simulink model "SWC_HALOUT_type"  (R2021b)
settings: Solver=FixedStepDiscrete  StartTime=0.0  StopTime=10.0  FixedStep=0.005  RelTol=1e-3
values from neighbouring files (symbols this model uses):
  DTC_10020B = Simulink.Parameter    [DTC_Constant_Definition.m]
  DTC_10020C = Simulink.Parameter    [DTC_Constant_Definition.m]
  DTC_10020D = Simulink.Parameter    [DTC_Constant_Definition.m]
  DTC_10020E = Simulink.Parameter    [DTC_Constant_Definition.m]
  DTC_100210 = Simulink.Parameter    [DTC_Constant_Definition.m]
  DTC_100211 = Simulink.Parameter    [DTC_Constant_Definition.m]
  DTC_100212 = Simulink.Parameter    [DTC_Constant_Definition.m]
  DTC_100213 = Simulink.Parameter    [DTC_Constant_Definition.m]
  DTC_100214 = Simulink.Parameter    [DTC_Constant_Definition.m]
  DTC_100215 = Simulink.Parameter    [DTC_Constant_Definition.m]
  DTC_100216 = Simulink.Parameter    [DTC_Constant_Definition.m]
  DTC_100217 = Simulink.Parameter    [DTC_Constant_Definition.m]
  DTC_100218 = Simulink.Parameter    [DTC_Constant_Definition.m]
  DTC_100219 = Simulink.Parameter    [DTC_Constant_Definition.m]
  DTC_10021A = Simulink.Parameter    [DTC_Constant_Definition.m]
  DTC_10021B = Simulink.Parameter    [DTC_Constant_Definition.m]
  DTC_10021C = Simulink.Parameter    [DTC_Constant_Definition.m]
  DTC_10021D = Simulink.Parameter    [DTC_Constant_Definition.m]
  DTC_10021E = Simulink.Parameter    [DTC_Constant_Definition.m]
  DTC_100220 = Simulink.Parameter    [DTC_Constant_Definition.m]
  DTC_100221 = Simulink.Parameter    [DTC_Constant_Definition.m]
  DTC_100223 = Simulink.Parameter    [DTC_Constant_Definition.m]
  DTC_100224 = Simulink.Parameter    [DTC_Constant_Definition.m]
  DTC_100225 = Simulink.Parameter    [DTC_Constant_Definition.m]
  DTC_100226 = Simulink.Parameter    [DTC_Constant_Definition.m]
  DTC_100227 = Simulink.Parameter    [DTC_Constant_Definition.m]
  DTC_100242 = Simulink.Parameter    [DTC_Constant_Definition.m]
  DTC_100243 = Simulink.Parameter    [DTC_Constant_Definition.m]
  DTC_100244 = Simulink.Parameter    [DTC_Constant_Definition.m]
  DTC_100247 = Simulink.Parameter    [DTC_Constant_Definition.m]
  DTC_100248 = Simulink.Parameter    [DTC_Constant_Definition.m]
  DTC_100249 = Simulink.Parameter    [DTC_Constant_Definition.m]
  DTC_100250 = Simulink.Parameter    [DTC_Constant_Definition.m]
  DTC_100251 = Simulink.Parameter    [DTC_Constant_Definition.m]
  DTC_100252 = Simulink.Parameter    [DTC_Constant_Definition.m]
  DTC_100A10 = Simulink.Parameter    [DTC_Constant_Definition.m]
  DTC_100A12 = Simulink.Parameter    [DTC_Constant_Definition.m]
  DTC_100A16 = Simulink.Parameter    [DTC_Constant_Definition.m]
  DTC_100A17 = Simulink.Parameter    [DTC_Constant_Definition.m]
  DTC_100A18 = Simulink.Parameter    [DTC_Constant_Definition.m]
  DTC_100A19 = Simulink.Parameter    [DTC_Constant_Definition.m]
  DTC_500B01 = Simulink.Parameter    [DTC_Constant_Definition.m]
  DTC_500B02 = Simulink.Parameter    [DTC_Constant_Definition.m]
  DTC_500B03 = Simulink.Parameter    [DTC_Constant_Definition.m]
  DTC_500B04 = Simulink.Parameter    [DTC_Constant_Definition.m]
  DTC_500B05 = Simulink.Parameter    [DTC_Constant_Definition.m]
  DTC_500B06 = Simulink.Parameter    [DTC_Constant_Definition.m]
  DTC_500B07 = Simulink.Parameter    [DTC_Constant_Definition.m]
  DTC_500B08 = Simulink.Parameter    [DTC_Constant_Definition.m]
  DTC_500B09 = Simulink.Parameter    [DTC_Constant_Definition.m]
  DTC_500B0A = Simulink.Parameter    [DTC_Constant_Definition.m]
  DTC_500B0B = Simulink.Parameter    [DTC_Constant_Definition.m]
  DTC_500B0C = Simulink.Parameter    [DTC_Constant_Definition.m]
  DTC_500B0D = Simulink.Parameter    [DTC_Constant_Definition.m]
  DTC_500B0E = Simulink.Parameter    [DTC_Constant_Definition.m]
  DTC_500B0F = Simulink.Parameter    [DTC_Constant_Definition.m]
  DTC_500B10 = Simulink.Parameter    [DTC_Constant_Definition.m]
  DTC_90021F = Simulink.Parameter    [DTC_Constant_Definition.m]
  DTC_90022F = Simulink.Parameter    [DTC_Constant_Definition.m]
  DTC_900253 = Simulink.Parameter    [DTC_Constant_Definition.m]
  DTC_900254 = Simulink.Parameter    [DTC_Constant_Definition.m]
  DTC_900301 = Simulink.Parameter    [DTC_Constant_Definition.m]
  DTC_900302 = Simulink.Parameter    [DTC_Constant_Definition.m]
  DTC_900303 = Simulink.Parameter    [DTC_Constant_Definition.m]
  DTC_900304 = Simulink.Parameter    [DTC_Constant_Definition.m]
  DTC_900305 = Simulink.Parameter    [DTC_Constant_Definition.m]
  DTC_900909 = Simulink.Parameter    [DTC_Constant_Definition.m]
  DTC_90090A = Simulink.Parameter    [DTC_Constant_Definition.m]
  DTC_90090B = Simulink.Parameter    [DTC_Constant_Definition.m]
  DTC_90090C = Simulink.Parameter    [DTC_Constant_Definition.m]
  DTC_90090D = Simulink.Parameter    [DTC_Constant_Definition.m]
  DTC_90090E = Simulink.Parameter    [DTC_Constant_Definition.m]
  DTC_90090F = Simulink.Parameter    [DTC_Constant_Definition.m]
  DTC_900910 = Simulink.Parameter    [DTC_Constant_Definition.m]
  DTC_900911 = Simulink.Parameter    [DTC_Constant_Definition.m]
  DTC_900912 = Simulink.Parameter    [DTC_Constant_Definition.m]
  DTC_900913 = Simulink.Parameter    [DTC_Constant_Definition.m]
  DTC_900914 = Simulink.Parameter    [DTC_Constant_Definition.m]
  DTC_C0288F = Simulink.Parameter    [DTC_Constant_Definition.m]
  DTC_C0378F = Simulink.Parameter    [DTC_Constant_Definition.m]
  DTC_C0468F = Simulink.Parameter    [DTC_Constant_Definition.m]
  DTC_C0558F = Simulink.Parameter    [DTC_Constant_Definition.m]
  DTC_C0648F = Simulink.Parameter    [DTC_Constant_Definition.m]
  DTC_C0808F = Simulink.Parameter    [DTC_Constant_Definition.m]
  DTC_D00201 = Simulink.Parameter    [DTC_Constant_Definition.m]
  DTC_D00202 = Simulink.Parameter    [DTC_Constant_Definition.m]
  DTC_D00203 = Simulink.Parameter    [DTC_Constant_Definition.m]
  DTC_D00204 = Simulink.Parameter    [DTC_Constant_Definition.m]
  DTC_D00205 = Simulink.Parameter    [DTC_Constant_Definition.m]
  DTC_D00206 = Simulink.Parameter    [DTC_Constant_Definition.m]
  DTC_D00207 = Simulink.Parameter    [DTC_Constant_Definition.m]
  DTC_D00208 = Simulink.Parameter    [DTC_Constant_Definition.m]
  DTC_D00209 = Simulink.Parameter    [DTC_Constant_Definition.m]
  DTC_D0020A = Simulink.Parameter    [DTC_Constant_Definition.m]
  DTC_D00228 = Simulink.Parameter    [DTC_Constant_Definition.m]
  DTC_D00229 = Simulink.Parameter    [DTC_Constant_Definition.m]
  DTC_D0022A = Simulink.Parameter    [DTC_Constant_Definition.m]
  DTC_D0022B = Simulink.Parameter    [DTC_Constant_Definition.m]
  DTC_D0022C = Simulink.Parameter    [DTC_Constant_Definition.m]
  DTC_D0022D = Simulink.Parameter    [DTC_Constant_Definition.m]
  DTC_D00230 = Simulink.Parameter    [DTC_Constant_Definition.m]
  DTC_D00231 = Simulink.Parameter    [DTC_Constant_Definition.m]
  DTC_D00232 = Simulink.Parameter    [DTC_Constant_Definition.m]
  DTC_D00234 = Simulink.Parameter    [DTC_Constant_Definition.m]
  DTC_D00235 = Simulink.Parameter    [DTC_Constant_Definition.m]
  DTC_D00236 = Simulink.Parameter    [DTC_Constant_Definition.m]
  DTC_D00237 = Simulink.Parameter    [DTC_Constant_Definition.m]
  DTC_D00238 = Simulink.Parameter    [DTC_Constant_Definition.m]
  DTC_D0023A = Simulink.Parameter    [DTC_Constant_Definition.m]
  DTC_D0023B = Simulink.Parameter    [DTC_Constant_Definition.m]
  DTC_D0023C = Simulink.Parameter    [DTC_Constant_Definition.m]
  DTC_D0023D = Simulink.Parameter    [DTC_Constant_Definition.m]
  DTC_D0023E = Simulink.Parameter    [DTC_Constant_Definition.m]
  DTC_D00240 = Simulink.Parameter    [DTC_Constant_Definition.m]
  DTC_D00241 = Simulink.Parameter    [DTC_Constant_Definition.m]
undefined symbols (not defined in the file or in its folder): DIDLen_APPD, DIDLen_APPE, DIDLen_APPPedalZP, DIDLen_APSFunConfig, DIDLen_AutoLock, DIDLen_AutoWipHSpdEN, DIDLen_CALID, DIDLen_CDEODT, DIDLen_CLRDIST, DIDLen_DKCBLESta, DIDLen_DKCKey, DIDLen_DKCSta, DIDLen_DoorNFCAnchorSta, DIDLen_DRLDis, DIDLen_DynoMode, DIDLen_ECUNAME, DIDLen_FDDKCCoordXY, DIDLen_FMHTimer, DIDLen_LFLowPresThre, DIDLen_LFSensorID, DIDLen_LIDAAnchorSta, DIDLen_LRLowPresThre, DIDLen_LRSensorID, DIDLen_MILDIST, DIDLen_NUMPSATRIPSFLTMEMCLR, DIDLen_NVMPedalZP, DIDLen_OBDReq, DIDLen_ODOMETER, DIDLen_PKE, DIDLen_ProtocolId, DIDLen_PSA, DIDLen_QTYPSATRIPS, DIDLen_RFLowPresThre, DIDLen_RFSensorID, DIDLen_RRLowPresThre, DIDLen_RRSensorID, DIDLen_RUNTM, DIDLen_SensorMode, DIDLen_TestGroup, DIDLen_TireSize, DIDLen_TPMSLearnSta, DIDLen_UIDSta, DIDLen_USSConfig, DIDLen_UWBAnchorSta, DIDLen_VIN, DIDLen_VSS, DIDLen_WhlPres, DIDLen_WhlSensorBattSta, DIDLen_WhlTmp, DIDLen_WipRLSCmdCutFilter, DIDLen_WipRLSCmdHoldFilter, DIDLen_XWDMode, DIDNum_APPD, DIDNum_APPE, DIDNum_APPPedalZP, DIDNum_APSFunConfig, DIDNum_AutoLock, DIDNum_AutoWipHSpdEN, DIDNum_CALID, DIDNum_CDEODT ... (+281)
libraries: simulink x213, FVT_lib x160, hdlsllib x6, hcu_lib x5, halout x1
(part 8 of 9)

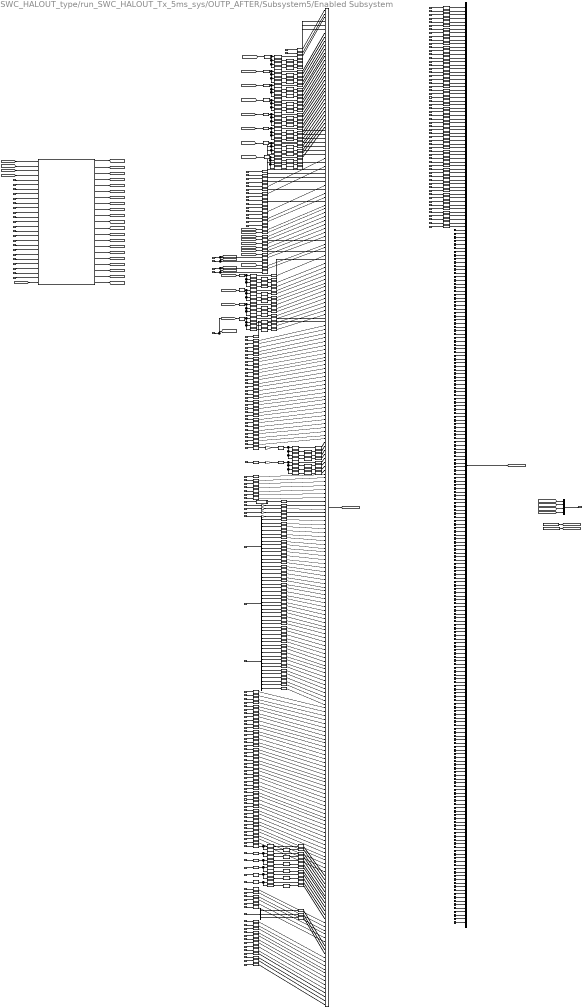
== system SWC_HALOUT_type/run_SWC_HALOUT_Tx_5ms_sys/OUTP_AFTER/Subsystem5/Enabled Subsystem ==
  VOUTP_AntitheftSta_enum : Inport
  VOUTP_DrivetrainSelect_enum : Inport  Port=2
  VOUTP_WriteChkLFID_raw : Inport  Port=3
  VOUTP_WriteChkRFID_raw : Inport  Port=4
  VOUTP_WriteChkLRID_raw : Inport  Port=5
  VOUTP_WriteChkRRID_raw : Inport  Port=6
  VOUTP_WriteChkfinLFID_raw : Inport  Port=7
  VOUTP_WriteChkfinRFID_raw : Inport  Port=8
  VOUTP_WriteChkfinLRID_raw : Inport  Port=9
  VOUTP_WriteChkfinRRID_raw : Inport  Port=10
  VOUTP_LFSensorFail_flg : Inport  Port=11
  VOUTP_RFSensorFail_flg : Inport  Port=12
  VOUTP_LRSensorFail_flg : Inport  Port=13
  VOUTP_RRSensorFail_flg : Inport  Port=14
  VOUTP_LFWheelPSW_raw8 : Inport  Port=15
  VOUTP_RFWheelPSW_raw8 : Inport  Port=16
  VOUTP_LRWheelPSW_raw8 : Inport  Port=17
  VOUTP_RRWheelPSW_raw8 : Inport  Port=18
  VOUTP_LFPindi_enum : Inport  Port=19
  VOUTP_RFPindi_enum : Inport  Port=20
  VOUTP_LRPindi_enum : Inport  Port=21
  VOUTP_RRPindi_enum : Inport  Port=22
  VOUTP_LFP20_raw8 : Inport  Port=23
  VOUTP_RFP20_raw8 : Inport  Port=24
  VOUTP_LRP20_raw8 : Inport  Port=25
  VOUTP_RRP20_raw8 : Inport  Port=26
  VOUTP_LFWheelPress_raw8 : Inport  Port=27
  VOUTP_RFWheelPress_raw8 : Inport  Port=28
  VOUTP_LRWheelPress_raw8 : Inport  Port=29
  VOUTP_RRWheelPress_raw8 : Inport  Port=30
  VOUTP_LFWheelTemp_C : Inport  Port=31
  VOUTP_RFWheelTemp_C : Inport  Port=32
  VOUTP_LRWheelTemp_C : Inport  Port=33
  VOUTP_RRWheelTemp_C : Inport  Port=34
  VOUTP_Flashchkdatavalid_enum : Inport  Port=35
  VOUTP_Flashdatavalid_enum : Inport  Port=36
  VOUTP_unlearnSfali_flg : Inport  Port=37
  VOUTP_unlearnSfailvalid_enum : Inport  Port=38
  VOUTP_Prepresstempvalid_enum : Inport  Port=39
  VOUTP_FlashS1ID_raw : Inport  Port=40
  VOUTP_FlashS2ID_raw : Inport  Port=41
  VOUTP_FlashS3ID_raw : Inport  Port=42
  VOUTP_FlashS41ID_raw : Inport  Port=43
  VOUTP_FlashIDvalid_enum : Inport  Port=44
  VOUTP_ACModeMem_enum : Inport  Port=45
  VOUTP_Face_flg : Inport  Port=46
  VOUTP_Foot_flg : Inport  Port=47
  VOUTP_Frost_flg : Inport  Port=48
  VOUTP_FaceM_flg : Inport  Port=49
  VOUTP_FootM_flg : Inport  Port=50
  VOUTP_CCUSyncSts_flg : Inport  Port=51
  VOUTP_ACForceOFF_flg : Inport  Port=52
  VOUTP_sigRecircSt_flg : Inport  Port=53
  VOUTP_RecAutoFlg_flg : Inport  Port=54
  VOUTP_AirIntenZone1M_enum : Inport  Port=55
  VOUTP_fdefog_flg : Inport  Port=56
  VOUTP_sigSetTempZon1St_C : Inport  Port=57
  VOUTP_sigSetTempZon2StM_C : Inport  Port=58
  VOUT_CountAlarm_enum : Inport  Port=59
  VOUTP_MFSWTri_flg : Inport  Port=60
  VOUTP_MirrorFlodPos_flg : Inport  Port=61
  VOUTP_FuelDoorPos_flg : Inport  Port=62
  VOUTP_LockSetting_flg : Inport  Port=63
  VOUTP_MFRDNBrightReq_pct : Inport  Port=64
  VOUTP_RoomLampMode_flg : Inport  Port=65
  VOUTP_WiperFixMode_flg : Inport  Port=66
  VOUTP_IVIPTGUSStaSW_flg : Inport  Port=67
  VOUTP_EAPS1MIN_pct : Inport  Port=68
  VOUTP_EAPS2MIN_pct : Inport  Port=69
  VOUTP_HoodSW_flg : Inport  Port=70
  VOUTP_TailgateSW_flg : Inport  Port=71
  VOUTP_CTDLockSW_flg : Inport  Port=72
  VOUTP_TailgateHDSW_flg : Inport  Port=73
  VOUTP_APMDoorControlSta_flg : Inport  Port=74
  VOUTP_fUnlockSingle_flg : Inport  Port=75
  VOUTP_SaveRegenMode_enum : Inport  Port=76
  VOUTP_AmbFunENFlash_enum : Inport  Port=77
  VOUTP_AmbWelENFlash_enum : Inport  Port=78
  VOUTP_AmbDimENFlash_enum : Inport  Port=79
  VOUTP_AmbLinkDriStaFlash_enum : Inport  Port=80
  VOUTP_AmbPwrWarnENFlash_enum : Inport  Port=81
  VOUTP_AmbODAENFlash_enum : Inport  Port=82
  VOUTP_AmbColorSta1_enum : Inport  Port=83
  VOUTP_AmbColorSta2_enum : Inport  Port=84
  VOUTP_AmbColorSta3_enum : Inport  Port=85
  VOUTP_AmbColorSta4_enum : Inport  Port=86
  VOUTP_AmbColorSta5_enum : Inport  Port=87
  VOUTP_AmbColorSta7_enum : Inport  Port=88
  VOUTP_AmbBrightnessSta1_enum : Inport  Port=89
  VOUTP_AmbBrightnessSta2_enum : Inport  Port=90
  VOUTP_AmbBrightnessSta3_enum : Inport  Port=91
  VOUTP_AmbBrightnessSta4_enum : Inport  Port=92
  VOUTP_AmbBrightnessSta5_enum : Inport  Port=93
  VOUTP_AmbBrightnessSta7_enum : Inport  Port=94
  VOUTP_TurnSwTimeSetSta123_enum : Inport  Port=95
  VOUTP_TurnSwTimeSetSta457_enum : Inport  Port=96
  VOUTP_FDCTHCAirIntZ3Sta_enum : Inport  Port=97
  VOUTP_FDCTHCREVentModeSta_enum : Inport  Port=98
  VOUTP_FDCTHCLEVentModeSta_enum : Inport  Port=99
  VOUTP_FDCTHCLEVentZSta_enum : Inport  Port=100
  VOUTP_FDCTHCCLEVentZSta_enum : Inport  Port=101
  VOUTP_FDCTHCREVentZSta_enum : Inport  Port=102
  VOUTP_FDCTHCCREVentZSta_enum : Inport  Port=103
  VOUTP_LVentEN_flg : Inport  Port=104
  VOUTP_FDCTHCLEVentYSta_enum : Inport  Port=105
  VOUTP_CLVentEN_flg : Inport  Port=106
  VOUTP_FDCTHCCLEVentYSta_enum : Inport  Port=107
  VOUTP_RVentEN_flg : Inport  Port=108
  VOUTP_FDCTHCREVentYSta_enum : Inport  Port=109
  VOUTP_CRVentEN_flg : Inport  Port=110
  VOUTP_FDCTHCCREVentYSta_enum : Inport  Port=111
  VOUTP_FDCFGSAirIntSta_enum : Inport  Port=112
  VOUTP_FDCFGSChSta_enum : Inport  Port=113
  VOUTP_FDCFGSIONSWSta_flg : Inport  Port=114
  VOUTP_WalkOutLkENFunSta_flg : Inport  Port=115
  VOUTP_WalkInUnLkENFunSta_flg : Inport  Port=116
  VOUTP_FollowMeENFunSta_flg : Inport  Port=117
  VOUTP_PTGUserHeight1_cnt : Inport  Port=118
  VOUTP_PTGUserHeight2_cnt : Inport  Port=119
  VOUTP_PTGUserHeight3_cnt : Inport  Port=120
  VOUTP_PTGUserHeight4_cnt : Inport  Port=121
  VOUTP_PTGUserHeight5_cnt : Inport  Port=122
  VOUTP_PTGUserHeight7_cnt : Inport  Port=123
  VOUTP_PTGOpenHeight12_enum : Inport  Port=124
  VOUTP_PTGOpenHeight34_enum : Inport  Port=125
  VOUTP_PTGOpenHeight57_enum : Inport  Port=126
  VOUTP_ACCLevelMem12_enum : Inport  Port=127
  VOUTP_ACCLevelMem34_enum : Inport  Port=128
  VOUTP_ACCLevelMem57_enum : Inport  Port=129
  VOUTP_AutoLockMem_enum : Inport  Port=130
  VOUTP_AutoUnlockMem_enum : Inport  Port=131
  VOUTP_ModelVersion_raw : Inport  Port=132
  VOUTP_ModelVersionChksum_raw : Inport  Port=133
  VOUTP_HMIKey1FuncSta_enum : Inport  Port=134
  VOUTP_HMIKey2FuncSta_enum : Inport  Port=135
  VOUTP_HMIKey3FuncSta_enum : Inport  Port=136
  VOUTP_HMIKey4FuncSta_enum : Inport  Port=137
  VOUTP_HMIKey5FuncSta_enum : Inport  Port=138
  VOUTP_HMIKey6FuncSta_enum : Inport  Port=139
  VOUTP_HMIKey7FuncSta_enum : Inport  Port=140
  VOUTP_HMIKey8FuncSta_enum : Inport  Port=141
  VOUTP_AutoWipHSpdENSta_flg : Inport  Port=142
  VOUTP_AirIntenZone1MSet2_enum : Inport  Port=143
  VOUTP_AirIntenZone1MSet3_enum : Inport  Port=144
  VOUTP_AirIntenZone1MSet4_enum : Inport  Port=145
  VOUTP_AirIntenZone1MSet5_enum : Inport  Port=146
  VOUTP_AirIntenZone1MSet7_enum : Inport  Port=147
  VOUTP_AirIntenZone3MSet2_enum : Inport  Port=148
  VOUTP_AirIntenZone3MSet3_enum : Inport  Port=149
  VOUTP_AirIntenZone3MSet4_enum : Inport  Port=150
  VOUTP_AirIntenZone3MSet5_enum : Inport  Port=151
  VOUTP_AirIntenZone3MSet7_enum : Inport  Port=152
  VOUTP_FDCFGSChStaSet457_enum : Inport  Port=153
  VOUTP_FDCFGSAirIntStaSet457_enum : Inport  Port=154
  VOUTP_LEVentModeStaSet457_enum : Inport  Port=155
  VOUTP_REVentModeStaSet457_enum : Inport  Port=156
  VOUTP_FDCTHCLEVentZStaSet2_enum : Inport  Port=157
  VOUTP_FDCTHCLEVentZStaSet3_enum : Inport  Port=158
  VOUTP_FDCTHCLEVentZStaSet4_enum : Inport  Port=159
  VOUTP_FDCTHCLEVentZStaSet5_enum : Inport  Port=160
  VOUTP_FDCTHCLEVentZStaSet7_enum : Inport  Port=161
  VOUTP_FDCTHCCLEVentZStaSet2_enum : Inport  Port=162
  VOUTP_FDCTHCCLEVentZStaSet3_enum : Inport  Port=163
  VOUTP_FDCTHCCLEVentZStaSet4_enum : Inport  Port=164
  VOUTP_FDCTHCCLEVentZStaSet5_enum : Inport  Port=165
  VOUTP_FDCTHCCLEVentZStaSet7_enum : Inport  Port=166
  VOUTP_FDCTHCREVentZStaSet2_enum : Inport  Port=167
  VOUTP_FDCTHCREVentZStaSet3_enum : Inport  Port=168
  VOUTP_FDCTHCREVentZStaSet4_enum : Inport  Port=169
  VOUTP_FDCTHCREVentZStaSet5_enum : Inport  Port=170
  VOUTP_FDCTHCREVentZStaSet7_enum : Inport  Port=171
  VOUTP_FDCTHCCREVentZStaSet2_enum : Inport  Port=172
  VOUTP_FDCTHCCREVentZStaSet3_enum : Inport  Port=173
  VOUTP_FDCTHCCREVentZStaSet4_enum : Inport  Port=174
  VOUTP_FDCTHCCREVentZStaSet5_enum : Inport  Port=175
  VOUTP_FDCTHCCREVentZStaSet7_enum : Inport  Port=176
  VOUTP_FDCTHCLEVentYStaSet2_enum : Inport  Port=177
  VOUTP_FDCTHCLEVentYStaSet3_enum : Inport  Port=178
  VOUTP_FDCTHCLEVentYStaSet4_enum : Inport  Port=179
  VOUTP_FDCTHCLEVentYStaSet5_enum : Inport  Port=180
  VOUTP_FDCTHCLEVentYStaSet7_enum : Inport  Port=181
  VOUTP_FDCTHCCLEVentYStaSet2_enum : Inport  Port=182
  VOUTP_FDCTHCCLEVentYStaSet3_enum : Inport  Port=183
  VOUTP_FDCTHCCLEVentYStaSet4_enum : Inport  Port=184
  VOUTP_FDCTHCCLEVentYStaSet5_enum : Inport  Port=185
  VOUTP_FDCTHCCLEVentYStaSet7_enum : Inport  Port=186
  VOUTP_FDCTHCREVentYStaSet2_enum : Inport  Port=187
  VOUTP_FDCTHCREVentYStaSet3_enum : Inport  Port=188
  VOUTP_FDCTHCREVentYStaSet4_enum : Inport  Port=189
  VOUTP_FDCTHCREVentYStaSet5_enum : Inport  Port=190
  VOUTP_FDCTHCREVentYStaSet7_enum : Inport  Port=191
  VOUTP_FDCTHCCREVentYStaSet2_enum : Inport  Port=192
  VOUTP_FDCTHCCREVentYStaSet3_enum : Inport  Port=193
  VOUTP_FDCTHCCREVentYStaSet4_enum : Inport  Port=194
  VOUTP_FDCTHCCREVentYStaSet5_enum : Inport  Port=195
  VOUTP_FDCTHCCREVentYStaSet7_enum : Inport  Port=196
  VOUTP_ACModeSet457_enum : Inport  Port=197
  VOUTP_SettempZon1Set2_enum : Inport  Port=198
  VOUTP_SettempZon1Set3_enum : Inport  Port=199
  VOUTP_SettempZon1Set4_enum : Inport  Port=200
  VOUTP_SettempZon1Set5_enum : Inport  Port=201
  VOUTP_SettempZon1Set7_enum : Inport  Port=202
  VOUTP_JudgeKeepUnlockZone_flg : Inport  Port=203
  VOUTP_CLWinLockDrStaMem_enum : Inport  Port=204
  BHAL_SYSTPMS_outputs : Inport  Port=205
  VHAL_RandomnumberY_raw1 : Inport  Port=206
  VHAL_RandomnumberY_raw2 : Inport  Port=207
  VHAL_RandomnumberY_raw3 : Inport  Port=208
  VHAL_RandomnumberY_raw4 : Inport  Port=209
  VHAL_RandomnumberY_raw5 : Inport  Port=210
  VHAL_RandomnumberY_raw6 : Inport  Port=211
  VHAL_RandomnumberY_raw7 : Inport  Port=212
  VHAL_RandomnumberY_raw8 : Inport  Port=213
  VHAL_funAuto_flg : Inport  Port=214
  VHAL_DiagDRLOFF_flg : Inport  Port=215
  VHAL_DiagFMHT_s : Inport  Port=216
  VHAL_DiagFLTC_mA : Inport  Port=217
  VHAL_DiagFRTC_mA : Inport  Port=218
  VHAL_DiagRLTC_mA : Inport  Port=219
  VHAL_DiagRRTC_mA : Inport  Port=220
  VHAL_USSConfig_raw8 : Inport  Port=221
  VHAL_TireSize_raw8 : Inport  Port=222
  VHAL_APSFunConfig_raw8 : Inport  Port=223
  BHAL_DIDGetData_raw : Inport  Port=224
  Bitwise AND{,4,8,14,16,22,26,30,32,36,40,44,48,52,56,58,60,62,64,66} (20 alike) : simulink/Logic and Bit Operations/Bitwise Operator  logicop=AND  UseBitMask=on  BitMask=bin2dec('00000000000000000000000011111111')  BitMaskRealWorld=Stored Integer
  Bitwise AND{1,5,9,15,17,23,27,31,33,37,41,45,49,53,57,59,61,63,65,67} (20 alike) : simulink/Logic and Bit Operations/Bitwise Operator  logicop=AND  UseBitMask=on  BitMask=bin2dec('00000000000000001111111100000000')  BitMaskRealWorld=Stored Integer
  Bitwise AND{2,6,10,12,18,20,24,28,34,38,42,46,50,54} (14 alike) : simulink/Logic and Bit Operations/Bitwise Operator  logicop=AND  UseBitMask=on  BitMask=bin2dec('00000000111111110000000000000000')  BitMaskRealWorld=Stored Integer
  Bitwise AND{3,7,11,13,19,21,25,29,35,39,43,47,51,55} (14 alike) : simulink/Logic and Bit Operations/Bitwise Operator  logicop=AND  UseBitMask=on  BitMask=bin2dec('11111111000000000000000000000000')  BitMaskRealWorld=Stored Integer
  Bus Selector2 : BusSelector  OutputSignals=VHAL_AutoWipHSpdEN_raw,VHAL_WipRLSCmdHoldFilter_raw,VHAL_WipRLSCmdCutFilter_raw
  Constant1 : Constant  Value=zeros(256,1)  OutDataTypeStr=uint8
  Constant2 : Constant  Value=zeros(256,1)  OutDataTypeStr=uint8
  Data Type Conversion{,1,5..13,15..18,20..23,25..27,29..32,34..37,39..40,42..106,108..111,113..116,118..121,123..126,128..130,132..235,237..239,241..242,244..245,247..248,250..251,253..329,779..787} (317 alike) : DataTypeConversion  OutDataTypeStr=uint8
  Data Type Conversion{4,14,19,24,28,33,38,41,107,112,117,122,127,131} (14 alike) : DataTypeConversion  OutDataTypeStr=uint32
  Data Type Conversion2 : DataTypeConversion  OutDataTypeStr=single
  Data Type Conversion{236,240,243,246,249,252} (6 alike) : DataTypeConversion  OutDataTypeStr=uint16
  Data Type Conversion3 : DataTypeConversion  OutDataTypeStr=single
  Demux : Demux  Outputs=16
  Demux1 : Demux  Outputs=16
  Demux2 : Demux  Outputs=16
  Gain{,1..3} (4 alike) : Gain  Gain=1/10
  Ground{2..195} (194 alike) : Ground
  Multiply : Gain  Gain=10000
  Multiply1 : Gain  Gain=10000
  Mux : Mux  Inputs=256
  Mux1 : Mux  Inputs=256
  Mux2 : Mux
  NVM1 : Subsystem
  Shift Arithmetic{,3,6,9,12,17,20,23..24,27,30,33,36,39,42..47} (20 alike) : ArithShift  BitShiftNumber=8  BitShiftDirection=Right
  Shift Arithmetic{1,4,7,10,13..14,18,21,25,28,31,34,37,40} (14 alike) : ArithShift  BitShiftNumber=16  BitShiftDirection=Right
  Shift Arithmetic{2,5,8,11,15..16,19,22,26,29,32,35,38,41} (14 alike) : ArithShift  BitShiftNumber=24  BitShiftDirection=Right
  Subsystem : Subsystem
  HAL_NvmWriteData_raw : Outport
  wires:
  Bitwise AND20/1 -> Shift Arithmetic14/1
  Shift Arithmetic4/1 -> Data Type Conversion12/1
  Data Type Conversion12/1 -> Mux/9
  Data Type Conversion30/1 -> Mux/24
  Shift Arithmetic23/1 -> Data Type Conversion40/1
  Bitwise AND1/1 -> Shift Arithmetic/1
  Bitwise AND11/1 -> Shift Arithmetic8/1
  Data Type Conversion5/1 -> Mux/21
  Bitwise AND17/1 -> Shift Arithmetic12/1
  Data Type Conversion32/1 -> Mux/30
  Data Type Conversion13/1 -> Mux/10
  Shift Arithmetic22/1 -> Data Type Conversion32/1
  Shift Arithmetic17/1 -> Data Type Conversion30/1
  Shift Arithmetic18/1 -> Data Type Conversion7/1
  Data Type Conversion14/1 -> Bitwise AND4/1, Bitwise AND7/1, Bitwise AND6/1, Bitwise AND5/1
  Bitwise AND26/1 -> Data Type Conversion29/1
  Data Type Conversion17/1 -> Mux/13
  Data Type Conversion25/1 -> Mux/15
  Data Type Conversion18/1 -> Mux/14
  Bitwise AND29/1 -> Shift Arithmetic19/1
  Shift Arithmetic8/1 -> Data Type Conversion18/1
  Data Type Conversion39/1 -> Mux/31
  Shift Arithmetic10/1 -> Data Type Conversion22/1
  Data Type Conversion6/1 -> Mux/22
  Bitwise AND28/1 -> Shift Arithmetic18/1
  Shift Arithmetic/1 -> Data Type Conversion9/1
  Data Type Conversion42/1 -> Mux/19
  Data Type Conversion11/1 -> Mux/6
  Shift Arithmetic19/1 -> Data Type Conversion27/1
  Data Type Conversion28/1 -> Bitwise AND26/1, Bitwise AND27/1, Bitwise AND28/1, Bitwise AND29/1
  Bitwise AND19/1 -> Shift Arithmetic22/1
  Bitwise AND27/1 -> Shift Arithmetic17/1
  Bitwise AND3/1 -> Shift Arithmetic2/1
  Data Type Conversion1/1 -> Mux/2
  Data Type Conversion26/1 -> Mux/16
  Bitwise AND23/1 -> Shift Arithmetic23/1
  Shift Arithmetic7/1 -> Data Type Conversion17/1
  Shift Arithmetic21/1 -> Data Type Conversion31/1
  Data Type Conversion8/1 -> Mux/3
  Data Type Conversion/1 -> Mux/1
  Bitwise AND10/1 -> Shift Arithmetic7/1
  Data Type Conversion37/1 -> Mux/34
  Data Type Conversion40/1 -> Mux/32
  Data Type Conversion36/1 -> Mux/33
  Bitwise AND/1 -> Data Type Conversion8/1
  Data Type Conversion20/1 -> Mux/11
  Data Type Conversion16/1 -> Mux/8
  Data Type Conversion21/1 -> Mux/12
  Data Type Conversion9/1 -> Mux/4
  Data Type Conversion10/1 -> Mux/5
  Data Type Conversion31/1 -> Mux/29
  Data Type Conversion15/1 -> Mux/7
  Data Type Conversion34/1 -> Mux/27
  Data Type Conversion35/1 -> Mux/28
  Data Type Conversion27/1 -> Mux/26
  Data Type Conversion29/1 -> Mux/23
  Data Type Conversion7/1 -> Mux/25
  Data Type Conversion22/1 -> Mux/17
  Data Type Conversion23/1 -> Mux/18
  Data Type Conversion43/1 -> Mux/20
  Data Type Conversion33/1 -> Bitwise AND19/1, Bitwise AND18/1, Bitwise AND31/1, Bitwise AND30/1
  Data Type Conversion41/1 -> Bitwise AND25/1, Bitwise AND24/1, Bitwise AND17/1, Bitwise AND16/1
  Bitwise AND30/1 -> Data Type Conversion34/1
  Bitwise AND24/1 -> Shift Arithmetic13/1
  Shift Arithmetic12/1 -> Data Type Conversion43/1
  Bitwise AND25/1 -> Shift Arithmetic16/1
  Bitwise AND18/1 -> Shift Arithmetic21/1
  Shift Arithmetic16/1 -> Data Type Conversion6/1
  Shift Arithmetic15/1 -> Data Type Conversion37/1
  Data Type Conversion38/1 -> Bitwise AND21/1, Bitwise AND20/1, Bitwise AND23/1, Bitwise AND22/1
  Bitwise AND31/1 -> Shift Arithmetic20/1
  Shift Arithmetic9/1 -> Data Type Conversion26/1
  Bitwise AND21/1 -> Shift Arithmetic15/1
  Data Type Conversion24/1 -> Bitwise AND14/1, Bitwise AND13/1, Bitwise AND12/1, Bitwise AND15/1
  Bitwise AND13/1 -> Shift Arithmetic11/1
  Bitwise AND9/1 -> Shift Arithmetic6/1
  Bitwise AND15/1 -> Shift Arithmetic9/1
  Bitwise AND12/1 -> Shift Arithmetic10/1
  Bitwise AND7/1 -> Shift Arithmetic5/1
  Shift Arithmetic2/1 -> Data Type Conversion11/1
  Shift Arithmetic1/1 -> Data Type Conversion10/1
  Data Type Conversion19/1 -> Bitwise AND11/1, Bitwise AND10/1, Bitwise AND9/1, Bitwise AND8/1
  Bitwise AND6/1 -> Shift Arithmetic4/1
  Bitwise AND5/1 -> Shift Arithmetic3/1
  Shift Arithmetic20/1 -> Data Type Conversion35/1
  Shift Arithmetic5/1 -> Data Type Conversion13/1
  Bitwise AND4/1 -> Data Type Conversion15/1
  Shift Arithmetic3/1 -> Data Type Conversion16/1
  Bitwise AND8/1 -> Data Type Conversion20/1
  Bitwise AND22/1 -> Data Type Conversion39/1
  Data Type Conversion4/1 -> Bitwise AND3/1, Bitwise AND2/1, Bitwise AND1/1, Bitwise AND/1
  Bitwise AND2/1 -> Shift Arithmetic1/1
  Shift Arithmetic11/1 -> Data Type Conversion23/1
  Shift Arithmetic14/1 -> Data Type Conversion36/1
  Shift Arithmetic13/1 -> Data Type Conversion5/1
  Bitwise AND14/1 -> Data Type Conversion25/1
  Shift Arithmetic6/1 -> Data Type Conversion21/1
  Bitwise AND16/1 -> Data Type Conversion42/1
  VOUTP_DrivetrainSelect_enum/1 -> Data Type Conversion1/1
  VOUTP_AntitheftSta_enum/1 -> Data Type Conversion/1
  Data Type Conversion66/1 -> Mux/57
  Data Type Conversion67/1 -> Mux/55
  VOUTP_ACModeMem_enum/1 -> Data Type Conversion81/1
  Data Type Conversion57/1 -> Mux/48
  VHAL_RandomnumberY_raw7/1 -> Data Type Conversion79/1
  VHAL_RandomnumberY_raw5/1 -> Data Type Conversion77/1
  VHAL_RandomnumberY_raw6/1 -> Data Type Conversion78/1
  Data Type Conversion72/1 -> Mux/62
  Data Type Conversion69/1 -> Mux/59
  VOUTP_Foot_flg/1 -> Data Type Conversion83/1
  [VHAL_NVMLRWheelPress_raw8] -> Data Type Conversion62/1
  VOUTP_LFSensorFail_flg/1 -> Data Type Conversion47/1
  [VHAL_NVMLFWheelPress_raw8] -> Data Type Conversion63/1
  VHAL_RandomnumberY_raw4/1 -> Data Type Conversion76/1
  VOUTP_Flashchkdatavalid_enum/1 -> [VOUTP_Flashchkdatavalid_enum], Data Type Conversion69/1
  Data Type Conversion63/1 -> Mux/51
  Data Type Conversion68/1 -> Mux/58
  Data Type Conversion51/1 -> Mux/39
  Data Type Conversion53/1 -> Mux/44
  VHAL_RandomnumberY_raw1/1 -> Data Type Conversion75/1
  Data Type Conversion48/1 -> Mux/38
  VOUTP_Face_flg/1 -> Data Type Conversion82/1
  VOUTP_LFP20_raw8/1 -> Data Type Conversion59/1
  VOUTP_CCUSyncSts_flg/1 -> Data Type Conversion87/1
  VHAL_RandomnumberY_raw3/1 -> Data Type Conversion74/1
  [VHAL_NVMRFWheelPress_raw8] -> Data Type Conversion61/1
  Data Type Conversion54/1 -> Mux/45
  Data Type Conversion47/1 -> Mux/35
  [VHAL_NVMunlearnSfali_flg] -> Data Type Conversion71/1
  VOUTP_RecAutoFlg_flg/1 -> Data Type Conversion90/1
  Data Type Conversion61/1 -> Mux/52
  VOUTP_fdefog_flg/1 -> Data Type Conversion92/1
  Data Type Conversion55/1 -> Mux/43
  VOUTP_sigRecircSt_flg/1 -> Data Type Conversion89/1
  Data Type Conversion52/1 -> Mux/42
  Data Type Conversion93/1 -> Mux/63
  Data Type Conversion56/1 -> Mux/46
  VOUTP_RFP20_raw8/1 -> Data Type Conversion57/1
  VOUTP_Prepresstempvalid_enum/1 -> [VOUTP_Prepresstempvalid_enum], Data Type Conversion93/1
  VOUTP_FaceM_flg/1 -> Data Type Conversion85/1
  Data Type Conversion58/1 -> Mux/49
  Data Type Conversion65/1 -> Mux/56
  VOUTP_RRPindi_enum/1 -> Data Type Conversion56/1
  VOUTP_FootM_flg/1 -> Data Type Conversion86/1
  Data Type Conversion50/1 -> Mux/41
  VOUTP_Flashdatavalid_enum/1 -> [VOUTP_Flashdatavalid_enum], Data Type Conversion70/1
  [VHAL_NVMRRWheelPress_raw8] -> Data Type Conversion64/1
  Data Type Conversion70/1 -> Mux/60
  [VHAL_NVMRRWheelTemp_C] -> Data Type Conversion68/1
  [VHAL_NVMLFWheelTemp_C] -> Data Type Conversion67/1
  VOUTP_AirIntenZone1M_enum/1 -> Data Type Conversion91/1
  Data Type Conversion64/1 -> Mux/54
  VOUTP_LRP20_raw8/1 -> Data Type Conversion58/1
  Data Type Conversion71/1 -> Mux/61
  VOUTP_RFPindi_enum/1 -> Data Type Conversion53/1
  VOUTP_RRP20_raw8/1 -> Data Type Conversion60/1
  Data Type Conversion49/1 -> Mux/40
  VOUTP_LRPindi_enum/1 -> Data Type Conversion54/1
  VOUTP_LFPindi_enum/1 -> Data Type Conversion55/1
  [VHAL_NVMLRWheelTemp_C] -> Data Type Conversion66/1
  Data Type Conversion62/1 -> Mux/53
  Data Type Conversion60/1 -> Mux/50
  Data Type Conversion59/1 -> Mux/47
  VOUTP_RRWheelPSW_raw8/1 -> Data Type Conversion52/1
  VHAL_RandomnumberY_raw2/1 -> Data Type Conversion73/1
  VOUTP_LRWheelPSW_raw8/1 -> Data Type Conversion50/1
  VHAL_RandomnumberY_raw8/1 -> Data Type Conversion80/1
  Data Type Conversion45/1 -> Mux/36
  VOUTP_ACForceOFF_flg/1 -> Data Type Conversion88/1
  Data Type Conversion46/1 -> Mux/37
  VOUTP_LFWheelPSW_raw8/1 -> Data Type Conversion51/1
  VOUTP_RRSensorFail_flg/1 -> Data Type Conversion48/1
  VOUTP_LRSensorFail_flg/1 -> Data Type Conversion46/1
  [VHAL_NVMRFWheelTemp_C] -> Data Type Conversion65/1
  VOUTP_RFWheelPSW_raw8/1 -> Data Type Conversion49/1
  VOUTP_RFSensorFail_flg/1 -> Data Type Conversion45/1
  VOUTP_Frost_flg/1 -> Data Type Conversion84/1
  Data Type Conversion134/1 -> Mux/120
  Data Type Conversion135/1 -> Mux/121
  Data Type Conversion136/1 -> Mux/122
  Data Type Conversion137/1 -> Mux/123
  Data Type Conversion255/1 -> Mux/235
  Mux/1 -> [HAL_NvmWriteData256BytesArray1_raw]
  NVM1/1(VHAL_NVMWriteChkLFID_raw) -> [VHAL_NVMWriteChkLFID_raw]
  VOUTP_WriteChkRFID_raw/1 -> NVM1/6(VOUTP_WriteChkRFID_raw)
  VOUTP_WriteChkLFID_raw/1 -> NVM1/5(VOUTP_WriteChkLFID_raw)
  VOUTP_WriteChkRRID_raw/1 -> NVM1/8(VOUTP_WriteChkRRID_raw)
  VOUTP_WriteChkLRID_raw/1 -> NVM1/7(VOUTP_WriteChkLRID_raw)
  [VOUTP_unlearnSfailvalid_enum] -> NVM1/3(VOUTP_unlearnSfailvalid_enum)
  [VOUTP_Flashchkdatavalid_enum] -> NVM1/1(VOUTP_Flashchkdatavalid_enum)
  [VOUTP_Prepresstempvalid_enum] -> NVM1/4(VOUTP_Prepresstempvalid_enum)
  [VOUTP_Flashdatavalid_enum] -> NVM1/2(VOUTP_Flashdatavalid_enum)
  VOUTP_unlearnSfailvalid_enum/1 -> Data Type Conversion72/1, [VOUTP_unlearnSfailvalid_enum]
  [VHAL_NVMWriteChkfinRRID_raw] -> Data Type Conversion38/1
  [VHAL_NVMWriteChkfinLRID_raw] -> Data Type Conversion33/1
  [VHAL_NVMWriteChkfinRFID_raw] -> Data Type Conversion28/1
  [VHAL_NVMWriteChkfinLFID_raw] -> Data Type Conversion41/1
  [VHAL_NVMWriteChkRRID_raw] -> Data Type Conversion24/1
  [VHAL_NVMWriteChkLRID_raw] -> Data Type Conversion19/1
  [VHAL_NVMWriteChkRFID_raw] -> Data Type Conversion14/1
  [VHAL_NVMWriteChkLFID_raw] -> Data Type Conversion4/1
  VOUT_CountAlarm_enum/1 -> Data Type Conversion99/1
  VOUTP_FuelDoorPos_flg/1 -> Data Type Conversion96/1
  VOUTP_LockSetting_flg/1 -> Data Type Conversion103/1
  VOUTP_WiperFixMode_flg/1 -> Data Type Conversion104/1
  VOUTP_MFRDNBrightReq_pct/1 -> Data Type Conversion100/1
  VOUTP_IVIPTGUSStaSW_flg/1 -> Data Type Conversion102/1
  VOUTP_RoomLampMode_flg/1 -> Data Type Conversion101/1
  VOUTP_MirrorFlodPos_flg/1 -> Data Type Conversion95/1
  VOUTP_sigSetTempZon2StM_C/1 -> Data Type Conversion98/1
  VOUTP_sigSetTempZon1St_C/1 -> Data Type Conversion97/1
  VOUTP_MFSWTri_flg/1 -> Data Type Conversion94/1
  VOUTP_WriteChkfinLRID_raw/1 -> NVM1/11(VOUTP_WriteChkfinLRID_raw)
  VOUTP_WriteChkfinRRID_raw/1 -> NVM1/12(VOUTP_WriteChkfinRRID_raw)
  VOUTP_WriteChkfinLFID_raw/1 -> NVM1/9(VOUTP_WriteChkfinLFID_raw)
  VOUTP_WriteChkfinRFID_raw/1 -> NVM1/10(VOUTP_WriteChkfinRFID_raw)
  VOUTP_LFWheelPress_raw8/1 -> NVM1/13(VOUTP_LFWheelPress_raw8)
  VOUTP_RFWheelPress_raw8/1 -> NVM1/14(VOUTP_RFWheelPress_raw8)
  VOUTP_RRWheelPress_raw8/1 -> NVM1/16(VOUTP_RRWheelPress_raw8)
  VOUTP_LRWheelPress_raw8/1 -> NVM1/15(VOUTP_LRWheelPress_raw8)
  VOUTP_LFWheelTemp_C/1 -> NVM1/17(VOUTP_LFWheelTemp_C)
  VOUTP_RFWheelTemp_C/1 -> NVM1/18(VOUTP_RFWheelTemp_C)
  VOUTP_LRWheelTemp_C/1 -> NVM1/19(VOUTP_LRWheelTemp_C)
  VOUTP_RRWheelTemp_C/1 -> NVM1/20(VOUTP_RRWheelTemp_C)
  VOUTP_unlearnSfali_flg/1 -> NVM1/21(VOUTP_unlearnSfali_flg)
  BHAL_SYSTPMS_outputs/1 -> NVM1/22(BHAL_SYSTPMS_outputs)
  VOUTP_FlashS41ID_raw/1 -> NVM1/26(VOUTP_FlashS4ID_raw)
  VOUTP_FlashS2ID_raw/1 -> NVM1/24(VOUTP_FlashS2ID_raw)
  VOUTP_FlashS1ID_raw/1 -> NVM1/23(VOUTP_FlashS1ID_raw)
  VOUTP_FlashS3ID_raw/1 -> NVM1/25(VOUTP_FlashS3ID_raw)
  [VOUTP_FlashIDvalid_enum] -> NVM1/27(VOUTP_FlashIDvalid_enum)
  VOUTP_FlashIDvalid_enum/1 -> Mux/80, [VOUTP_FlashIDvalid_enum]
  Shift Arithmetic32/1 -> Data Type Conversion116/1
  Bitwise AND35/1 -> Shift Arithmetic26/1
  Shift Arithmetic29/1 -> Data Type Conversion111/1
  Bitwise AND43/1 -> Shift Arithmetic32/1
  Bitwise AND33/1 -> Shift Arithmetic24/1
  Bitwise AND41/1 -> Shift Arithmetic30/1
  [VHAL_NVMFlashS4ID_raw] -> Data Type Conversion122/1
  Shift Arithmetic24/1 -> Data Type Conversion109/1
  Data Type Conversion107/1 -> Bitwise AND35/1, Bitwise AND34/1, Bitwise AND33/1, Bitwise AND32/1
  Shift Arithmetic33/1 -> Data Type Conversion124/1
  Shift Arithmetic34/1 -> Data Type Conversion120/1
  Data Type Conversion117/1 -> Bitwise AND43/1, Bitwise AND42/1, Bitwise AND41/1, Bitwise AND40/1
  Bitwise AND36/1 -> Data Type Conversion113/1
  Bitwise AND40/1 -> Data Type Conversion118/1
  Shift Arithmetic27/1 -> Data Type Conversion114/1
  Bitwise AND32/1 -> Data Type Conversion108/1
  Bitwise AND37/1 -> Shift Arithmetic27/1
  Data Type Conversion122/1 -> Bitwise AND47/1, Bitwise AND46/1, Bitwise AND45/1, Bitwise AND44/1
  Shift Arithmetic26/1 -> Data Type Conversion106/1
  Data Type Conversion112/1 -> Bitwise AND39/1, Bitwise AND38/1, Bitwise AND37/1, Bitwise AND36/1
  Bitwise AND39/1 -> Shift Arithmetic29/1
  Bitwise AND47/1 -> Shift Arithmetic35/1
  Bitwise AND44/1 -> Data Type Conversion123/1
  Bitwise AND46/1 -> Shift Arithmetic34/1
  [VHAL_NVMFlashS3ID_raw] -> Data Type Conversion117/1
  Shift Arithmetic30/1 -> Data Type Conversion119/1
  Bitwise AND34/1 -> Shift Arithmetic25/1
  Shift Arithmetic28/1 -> Data Type Conversion110/1
  Bitwise AND38/1 -> Shift Arithmetic28/1
  Bitwise AND45/1 -> Shift Arithmetic33/1
  [VHAL_NVMFlashS2ID_raw] -> Data Type Conversion112/1
  Shift Arithmetic25/1 -> Data Type Conversion105/1
  Shift Arithmetic35/1 -> Data Type Conversion121/1
  Shift Arithmetic31/1 -> Data Type Conversion115/1
  Bitwise AND42/1 -> Shift Arithmetic31/1
  [VHAL_NVMFlashS1ID_raw] -> Data Type Conversion107/1
  Data Type Conversion109/1 -> Mux/65
  Data Type Conversion105/1 -> Mux/66
  Data Type Conversion106/1 -> Mux/67
  Data Type Conversion114/1 -> Mux/69
  Data Type Conversion110/1 -> Mux/70
  Data Type Conversion111/1 -> Mux/71
  Data Type Conversion119/1 -> Mux/73
  Data Type Conversion115/1 -> Mux/74
  Data Type Conversion116/1 -> Mux/75
  Data Type Conversion124/1 -> Mux/77
  Data Type Conversion120/1 -> Mux/78
  Data Type Conversion121/1 -> Mux/79
  Data Type Conversion108/1 -> Mux/64
  Data Type Conversion113/1 -> Mux/68
  Data Type Conversion118/1 -> Mux/72
  Data Type Conversion123/1 -> Mux/76
  Data Type Conversion75/1 -> Mux/81
  Data Type Conversion73/1 -> Mux/82
  Data Type Conversion74/1 -> Mux/83
  Data Type Conversion76/1 -> Mux/84
  Data Type Conversion77/1 -> Mux/85
  Data Type Conversion78/1 -> Mux/86
  Data Type Conversion79/1 -> Mux/87
  Data Type Conversion80/1 -> Mux/88
  Data Type Conversion81/1 -> Mux/89
  Data Type Conversion82/1 -> Mux/90
  Data Type Conversion83/1 -> Mux/91
  Data Type Conversion84/1 -> Mux/92
  Data Type Conversion85/1 -> Mux/93
  Data Type Conversion86/1 -> Mux/94
  Data Type Conversion87/1 -> Mux/95
  Data Type Conversion88/1 -> Mux/96
  Data Type Conversion89/1 -> Mux/97
  Data Type Conversion90/1 -> Mux/98
  Data Type Conversion91/1 -> Mux/99
  Data Type Conversion92/1 -> Mux/100
  Data Type Conversion97/1 -> Mux/101
  Data Type Conversion98/1 -> Mux/102
  Data Type Conversion99/1 -> Mux/103
  Data Type Conversion94/1 -> Mux/104
  Data Type Conversion95/1 -> Mux/105
  Data Type Conversion96/1 -> Mux/106
  Data Type Conversion103/1 -> Mux/107
  Data Type Conversion100/1 -> Mux/108
  Data Type Conversion101/1 -> Mux/109
  Data Type Conversion104/1 -> Mux/110
  Data Type Conversion102/1 -> Mux/111
  NVM1/21(VHAL_NVMFlashS4ID_raw) -> [VHAL_NVMFlashS4ID_raw]
  NVM1/2(VHAL_NVMWriteChkRFID_raw) -> [VHAL_NVMWriteChkRFID_raw]
  NVM1/3(VHAL_NVMWriteChkLRID_raw) -> [VHAL_NVMWriteChkLRID_raw]
  NVM1/4(VHAL_NVMWriteChkRRID_raw) -> [VHAL_NVMWriteChkRRID_raw]
  NVM1/5(VHAL_NVMWriteChkfinLFID_raw) -> [VHAL_NVMWriteChkfinLFID_raw]
  NVM1/6(VHAL_NVMWriteChkfinRFID_raw) -> [VHAL_NVMWriteChkfinRFID_raw]
  NVM1/7(VHAL_NVMWriteChkfinLRID_raw) -> [VHAL_NVMWriteChkfinLRID_raw]
  NVM1/8(VHAL_NVMWriteChkfinRRID_raw) -> [VHAL_NVMWriteChkfinRRID_raw]
  NVM1/9(VHAL_NVMunlearnSfali_flg) -> [VHAL_NVMunlearnSfali_flg]
  NVM1/10(VHAL_NVMLFWheelPress_raw8) -> [VHAL_NVMLFWheelPress_raw8]
  NVM1/11(VHAL_NVMRFWheelPress_raw8) -> [VHAL_NVMRFWheelPress_raw8]
  NVM1/12(VHAL_NVMLRWheelPress_raw8) -> [VHAL_NVMLRWheelPress_raw8]
  NVM1/13(VHAL_NVMRRWheelPress_raw8) -> [VHAL_NVMRRWheelPress_raw8]
  NVM1/14(VHAL_NVMLFWheelTemp_C) -> [VHAL_NVMLFWheelTemp_C]
  NVM1/15(VHAL_NVMRFWheelTemp_C) -> [VHAL_NVMRFWheelTemp_C]
  NVM1/16(VHAL_NVMLRWheelTemp_C) -> [VHAL_NVMLRWheelTemp_C]
  NVM1/17(VHAL_NVMRRWheelTemp_C) -> [VHAL_NVMRRWheelTemp_C]
  NVM1/18(VHAL_NVMFlashS1ID_raw) -> [VHAL_NVMFlashS1ID_raw]
  NVM1/19(VHAL_NVMFlashS2ID_raw) -> [VHAL_NVMFlashS2ID_raw]
  NVM1/20(VHAL_NVMFlashS3ID_raw) -> [VHAL_NVMFlashS3ID_raw]
  VOUTP_EAPS1MIN_pct/1 -> Data Type Conversion2/1
  VOUTP_EAPS2MIN_pct/1 -> Data Type Conversion3/1
  Multiply/1 -> Data Type Conversion127/1
  Data Type Conversion126/1 -> Mux/115
  Data Type Conversion129/1 -> Mux/113
  Data Type Conversion125/1 -> Mux/114
  Shift Arithmetic37/1 -> Data Type Conversion125/1
  Shift Arithmetic38/1 -> Data Type Conversion126/1
  Data Type Conversion128/1 -> Mux/112
  Bitwise AND48/1 -> Data Type Conversion128/1
  Bitwise AND49/1 -> Shift Arithmetic36/1
  Data Type Conversion127/1 -> Bitwise AND51/1, Bitwise AND50/1, Bitwise AND49/1, Bitwise AND48/1
  Shift Arithmetic36/1 -> Data Type Conversion129/1
  Bitwise AND51/1 -> Shift Arithmetic38/1
  Bitwise AND50/1 -> Shift Arithmetic37/1
  Data Type Conversion2/1 -> Multiply/1
  Bitwise AND54/1 -> Shift Arithmetic40/1
  Bitwise AND55/1 -> Shift Arithmetic41/1
  Shift Arithmetic39/1 -> Data Type Conversion133/1
  Data Type Conversion131/1 -> Bitwise AND52/1, Bitwise AND53/1, Bitwise AND54/1, Bitwise AND55/1
  Bitwise AND53/1 -> Shift Arithmetic39/1
  Bitwise AND52/1 -> Data Type Conversion132/1
  Shift Arithmetic41/1 -> Data Type Conversion130/1
  Shift Arithmetic40/1 -> Data Type Conversion44/1
  Multiply1/1 -> Data Type Conversion131/1
  Data Type Conversion132/1 -> Mux/116
  Data Type Conversion133/1 -> Mux/117
  Data Type Conversion44/1 -> Mux/118
  Data Type Conversion130/1 -> Mux/119
  Data Type Conversion3/1 -> Multiply1/1
  VOUTP_HoodSW_flg/1 -> Data Type Conversion134/1
  VOUTP_TailgateHDSW_flg/1 -> Data Type Conversion137/1
  VOUTP_CTDLockSW_flg/1 -> Data Type Conversion136/1
  VOUTP_TailgateSW_flg/1 -> Data Type Conversion135/1
  VOUTP_APMDoorControlSta_flg/1 -> Data Type Conversion138/1
  Data Type Conversion138/1 -> Mux/124
  VHAL_funAuto_flg/1 -> Data Type Conversion139/1
  VHAL_DiagDRLOFF_flg/1 -> Data Type Conversion140/1
  Data Type Conversion139/1 -> Mux/125
  Data Type Conversion140/1 -> Mux/126
  Data Type Conversion141/1 -> Mux/127
  Data Type Conversion142/1 -> Mux/128
  Data Type Conversion143/1 -> Mux/129
  Data Type Conversion144/1 -> Mux/130
  Data Type Conversion145/1 -> Mux/131
  Demux/1 -> Data Type Conversion146/1
  Demux/2 -> Data Type Conversion147/1
  Demux/3 -> Data Type Conversion148/1
  Demux/4 -> Data Type Conversion149/1
  Demux/5 -> Data Type Conversion150/1
  Demux/6 -> Data Type Conversion151/1
  Demux/7 -> Data Type Conversion152/1
  Demux/8 -> Data Type Conversion153/1
  VHAL_USSConfig_raw8/1 -> Demux/1
  Data Type Conversion146/1 -> Mux/132
  Data Type Conversion147/1 -> Mux/133
  Data Type Conversion148/1 -> Mux/134
  Data Type Conversion149/1 -> Mux/135
  Data Type Conversion150/1 -> Mux/136
  Data Type Conversion151/1 -> Mux/137
  Data Type Conversion152/1 -> Mux/138
  Data Type Conversion153/1 -> Mux/139
  Demux/16 -> Data Type Conversion161/1
  Demux/15 -> Data Type Conversion160/1
  Demux/14 -> Data Type Conversion159/1
  Demux/13 -> Data Type Conversion158/1
  Demux/12 -> Data Type Conversion157/1
  Demux/11 -> Data Type Conversion156/1
  Demux/10 -> Data Type Conversion155/1
  Demux/9 -> Data Type Conversion154/1
  Data Type Conversion154/1 -> Mux/140
  Data Type Conversion155/1 -> Mux/141
  Data Type Conversion156/1 -> Mux/142
  Data Type Conversion157/1 -> Mux/143
  Data Type Conversion158/1 -> Mux/144
  Data Type Conversion159/1 -> Mux/145
  Data Type Conversion160/1 -> Mux/146
  Data Type Conversion161/1 -> Mux/147
  Data Type Conversion177/1 -> Mux/163
  Data Type Conversion176/1 -> Mux/162
  Data Type Conversion175/1 -> Mux/161
  Data Type Conversion174/1 -> Mux/160
  Data Type Conversion173/1 -> Mux/159
  Data Type Conversion172/1 -> Mux/158
  Data Type Conversion171/1 -> Mux/157
  Data Type Conversion170/1 -> Mux/156
  Demux1/9 -> Data Type Conversion170/1
  Demux1/10 -> Data Type Conversion171/1
  Demux1/11 -> Data Type Conversion172/1
  Demux1/12 -> Data Type Conversion173/1
  Demux1/13 -> Data Type Conversion174/1
  Demux1/14 -> Data Type Conversion175/1
  Demux1/15 -> Data Type Conversion176/1
  Demux1/16 -> Data Type Conversion177/1
  Data Type Conversion169/1 -> Mux/155
  Data Type Conversion168/1 -> Mux/154
  Data Type Conversion167/1 -> Mux/153
  Data Type Conversion166/1 -> Mux/152
  Data Type Conversion165/1 -> Mux/151
  Data Type Conversion164/1 -> Mux/150
  Data Type Conversion163/1 -> Mux/149
  Data Type Conversion162/1 -> Mux/148
  VHAL_TireSize_raw8/1 -> Demux1/1
  Demux1/8 -> Data Type Conversion169/1
  Demux1/7 -> Data Type Conversion168/1
  Demux1/6 -> Data Type Conversion167/1
  Demux1/5 -> Data Type Conversion166/1
  Demux1/4 -> Data Type Conversion165/1
  Demux1/3 -> Data Type Conversion164/1
  Demux1/2 -> Data Type Conversion163/1
  Demux1/1 -> Data Type Conversion162/1
  Demux2/1 -> Data Type Conversion178/1
  Demux2/2 -> Data Type Conversion179/1
  Demux2/3 -> Data Type Conversion180/1
  Demux2/4 -> Data Type Conversion181/1
  Demux2/5 -> Data Type Conversion182/1
  Demux2/6 -> Data Type Conversion183/1
  Demux2/7 -> Data Type Conversion184/1
  Demux2/8 -> Data Type Conversion185/1
  VHAL_APSFunConfig_raw8/1 -> Demux2/1
  Data Type Conversion178/1 -> Mux/164
  Data Type Conversion179/1 -> Mux/165
  Data Type Conversion180/1 -> Mux/166
  Data Type Conversion181/1 -> Mux/167
  Data Type Conversion182/1 -> Mux/168
  Data Type Conversion183/1 -> Mux/169
  Data Type Conversion184/1 -> Mux/170
  Data Type Conversion185/1 -> Mux/171
  Demux2/16 -> Data Type Conversion193/1
  Demux2/15 -> Data Type Conversion192/1
  Demux2/14 -> Data Type Conversion191/1
  Demux2/13 -> Data Type Conversion190/1
  Demux2/12 -> Data Type Conversion189/1
  Demux2/11 -> Data Type Conversion188/1
  Demux2/10 -> Data Type Conversion187/1
  Demux2/9 -> Data Type Conversion186/1
  Data Type Conversion186/1 -> Mux/172
  Data Type Conversion187/1 -> Mux/173
  Data Type Conversion188/1 -> Mux/174
  Data Type Conversion189/1 -> Mux/175
  Data Type Conversion190/1 -> Mux/176
  Data Type Conversion191/1 -> Mux/177
  Data Type Conversion192/1 -> Mux/178
  Data Type Conversion193/1 -> Mux/179
  VOUTP_fUnlockSingle_flg/1 -> Data Type Conversion194/1
  Data Type Conversion194/1 -> Mux/180
  Gain3/1 -> Data Type Conversion145/1
  Gain2/1 -> Data Type Conversion144/1
  Gain1/1 -> Data Type Conversion143/1
  Gain/1 -> Data Type Conversion142/1
  Subsystem/1(Out1) -> Data Type Conversion141/1
  VHAL_DiagFMHT_s/1 -> Subsystem/1(VOUTP_DiagFMHT_s)
  VHAL_DiagFRTC_mA/1 -> Gain1/1
  VHAL_DiagRLTC_mA/1 -> Gain2/1
  VHAL_DiagRRTC_mA/1 -> Gain3/1
  VHAL_DiagFLTC_mA/1 -> Gain/1
  VOUTP_SaveRegenMode_enum/1 -> Data Type Conversion195/1
  Data Type Conversion195/1 -> Mux/181
  Data Type Conversion212/1 -> Mux/198
  VOUTP_AmbPwrWarnENFlash_enum/1 -> Data Type Conversion200/1
  Data Type Conversion197/1 -> Mux/183
  Data Type Conversion199/1 -> Mux/185
  VOUTP_AmbColorSta5_enum/1 -> Data Type Conversion206/1
  VOUTP_AmbBrightnessSta1_enum/1 -> Data Type Conversion208/1
  VOUTP_AmbBrightnessSta3_enum/1 -> Data Type Conversion210/1
  Data Type Conversion213/1 -> Mux/199
  Data Type Conversion196/1 -> Mux/182
  Data Type Conversion202/1 -> Mux/188
  Data Type Conversion200/1 -> Mux/186
  VOUTP_AmbBrightnessSta2_enum/1 -> Data Type Conversion209/1
  Data Type Conversion209/1 -> Mux/195
  Data Type Conversion201/1 -> Mux/187
  VOUTP_AmbColorSta3_enum/1 -> Data Type Conversion204/1
  VOUTP_AmbColorSta1_enum/1 -> Data Type Conversion202/1
  VOUTP_AmbBrightnessSta7_enum/1 -> Data Type Conversion213/1
  VOUTP_AmbColorSta4_enum/1 -> Data Type Conversion205/1
  VOUTP_AmbODAENFlash_enum/1 -> Data Type Conversion201/1
  VOUTP_AmbLinkDriStaFlash_enum/1 -> Data Type Conversion199/1
  VOUTP_AmbFunENFlash_enum/1 -> Data Type Conversion196/1
  Data Type Conversion204/1 -> Mux/190
  Data Type Conversion203/1 -> Mux/189
  VOUTP_AmbDimENFlash_enum/1 -> Data Type Conversion198/1
  VOUTP_AmbColorSta2_enum/1 -> Data Type Conversion203/1
  VOUTP_AmbColorSta7_enum/1 -> Data Type Conversion207/1
  Data Type Conversion208/1 -> Mux/194
  VOUTP_AmbWelENFlash_enum/1 -> Data Type Conversion197/1
  Data Type Conversion205/1 -> Mux/191
  VOUTP_AmbBrightnessSta4_enum/1 -> Data Type Conversion211/1
  Data Type Conversion207/1 -> Mux/193
  Data Type Conversion211/1 -> Mux/197
  Data Type Conversion210/1 -> Mux/196
  Data Type Conversion206/1 -> Mux/192
  VOUTP_AmbBrightnessSta5_enum/1 -> Data Type Conversion212/1
  Data Type Conversion198/1 -> Mux/184
  VOUTP_FDCTHCLEVentYSta_enum/1 -> Data Type Conversion224/1
  Data Type Conversion232/1 -> Mux/218
  VOUTP_LVentEN_flg/1 -> Data Type Conversion223/1
  Data Type Conversion233/1 -> Mux/219
  VOUTP_FDCTHCCLEVentYSta_enum/1 -> Data Type Conversion226/1
  Data Type Conversion231/1 -> Mux/217
  Data Type Conversion224/1 -> Mux/210
  VOUTP_FDCTHCLEVentZSta_enum/1 -> Data Type Conversion219/1
  VOUTP_CRVentEN_flg/1 -> Data Type Conversion229/1
  VOUTP_FDCFGSIONSWSta_flg/1 -> Data Type Conversion233/1
  Data Type Conversion227/1 -> Mux/213
  VOUTP_FDCFGSAirIntSta_enum/1 -> Data Type Conversion231/1
  VOUTP_FDCFGSChSta_enum/1 -> Data Type Conversion232/1
  VOUTP_RVentEN_flg/1 -> Data Type Conversion227/1
  VOUTP_FDCTHCCREVentYSta_enum/1 -> Data Type Conversion230/1
  VOUTP_FDCTHCCREVentZSta_enum/1 -> Data Type Conversion222/1
  VOUTP_FDCTHCCLEVentZSta_enum/1 -> Data Type Conversion220/1
  Data Type Conversion217/1 -> Mux/203
  VOUTP_FDCTHCREVentModeSta_enum/1 -> Data Type Conversion217/1
  Data Type Conversion214/1 -> Mux/200
  VOUTP_TurnSwTimeSetSta457_enum/1 -> Data Type Conversion215/1
  VOUTP_FDCTHCLEVentModeSta_enum/1 -> Data Type Conversion218/1
  Data Type Conversion230/1 -> Mux/216
  VOUTP_CLVentEN_flg/1 -> Data Type Conversion225/1
  Data Type Conversion215/1 -> Mux/201
  VOUTP_FDCTHCREVentZSta_enum/1 -> Data Type Conversion221/1
  VOUTP_FDCTHCREVentYSta_enum/1 -> Data Type Conversion228/1
  VOUTP_TurnSwTimeSetSta123_enum/1 -> Data Type Conversion214/1
  Data Type Conversion221/1 -> Mux/207
  Data Type Conversion218/1 -> Mux/204
  Data Type Conversion219/1 -> Mux/205
  Data Type Conversion223/1 -> Mux/209
  Data Type Conversion226/1 -> Mux/212
  Data Type Conversion229/1 -> Mux/215
  Data Type Conversion222/1 -> Mux/208
  Data Type Conversion220/1 -> Mux/206
  VOUTP_FDCTHCAirIntZ3Sta_enum/1 -> Data Type Conversion216/1
  Data Type Conversion225/1 -> Mux/211
  Data Type Conversion228/1 -> Mux/214
  Data Type Conversion216/1 -> Mux/202
  VOUTP_WalkOutLkENFunSta_flg/1 -> Data Type Conversion234/1
  VOUTP_WalkInUnLkENFunSta_flg/1 -> Data Type Conversion235/1
  VOUTP_FollowMeENFunSta_flg/1 -> Data Type Conversion237/1
  Data Type Conversion234/1 -> Mux/220
  Data Type Conversion235/1 -> Mux/221
  Data Type Conversion237/1 -> Mux/222
  Data Type Conversion236/1 -> Bitwise AND57/1, Bitwise AND56/1
  Shift Arithmetic42/1 -> Data Type Conversion239/1
  Bitwise AND56/1 -> Data Type Conversion238/1
  Bitwise AND57/1 -> Shift Arithmetic42/1
  Data Type Conversion238/1 -> Mux/223
  Data Type Conversion239/1 -> Mux/224
  Bitwise AND59/1 -> Shift Arithmetic43/1
  Bitwise AND58/1 -> Data Type Conversion241/1
  Shift Arithmetic43/1 -> Data Type Conversion242/1
  Data Type Conversion240/1 -> Bitwise AND58/1, Bitwise AND59/1
  Data Type Conversion243/1 -> Bitwise AND61/1, Bitwise AND60/1
  Shift Arithmetic44/1 -> Data Type Conversion245/1
  Bitwise AND60/1 -> Data Type Conversion244/1
  Bitwise AND61/1 -> Shift Arithmetic44/1
  Bitwise AND67/1 -> Shift Arithmetic47/1
  Bitwise AND66/1 -> Data Type Conversion253/1
  Shift Arithmetic47/1 -> Data Type Conversion254/1
  Data Type Conversion252/1 -> Bitwise AND66/1, Bitwise AND67/1
  Data Type Conversion249/1 -> Bitwise AND65/1, Bitwise AND64/1
  Shift Arithmetic46/1 -> Data Type Conversion251/1
  Bitwise AND64/1 -> Data Type Conversion250/1
  Bitwise AND65/1 -> Shift Arithmetic46/1
  Bitwise AND63/1 -> Shift Arithmetic45/1
  Bitwise AND62/1 -> Data Type Conversion247/1
  Shift Arithmetic45/1 -> Data Type Conversion248/1
  Data Type Conversion246/1 -> Bitwise AND62/1, Bitwise AND63/1
  Data Type Conversion241/1 -> Mux/225
  Data Type Conversion242/1 -> Mux/226
  Data Type Conversion244/1 -> Mux/227
  Data Type Conversion245/1 -> Mux/228
  Data Type Conversion247/1 -> Mux/229
  Data Type Conversion248/1 -> Mux/230
  Data Type Conversion250/1 -> Mux/231
  Data Type Conversion251/1 -> Mux/232
  Data Type Conversion253/1 -> Mux/233
  Data Type Conversion254/1 -> Mux/234
  VOUTP_PTGUserHeight1_cnt/1 -> Data Type Conversion236/1
  VOUTP_PTGUserHeight2_cnt/1 -> Data Type Conversion240/1
  VOUTP_PTGUserHeight3_cnt/1 -> Data Type Conversion243/1
  VOUTP_PTGUserHeight4_cnt/1 -> Data Type Conversion246/1
  VOUTP_PTGUserHeight5_cnt/1 -> Data Type Conversion249/1
  VOUTP_PTGUserHeight7_cnt/1 -> Data Type Conversion252/1
  VOUTP_PTGOpenHeight12_enum/1 -> Data Type Conversion255/1
  VOUTP_PTGOpenHeight34_enum/1 -> Data Type Conversion256/1
  VOUTP_PTGOpenHeight57_enum/1 -> Data Type Conversion257/1
  Data Type Conversion256/1 -> Mux/236
  Data Type Conversion257/1 -> Mux/237
  Data Type Conversion260/1 -> Mux/243
  Data Type Conversion262/1 -> Mux/245
  Bus Selector2/3 -> Data Type Conversion260/1  "<VHAL_WipRLSCmdCutFilter_raw>"
  Data Type Conversion261/1 -> Mux/244
  BHAL_DIDGetData_raw/1 -> Bus Selector2/1
  VOUTP_AutoLockMem_enum/1 -> Data Type Conversion261/1
  Data Type Conversion259/1 -> Mux/242
  Data Type Conversion258/1 -> Mux/241
  Bus Selector2/1 -> Data Type Conversion258/1  "<VHAL_AutoWipHSpdEN_raw>"
  VOUTP_AutoUnlockMem_enum/1 -> Data Type Conversion262/1
  Bus Selector2/2 -> Data Type Conversion259/1  "<VHAL_WipRLSCmdHoldFilter_raw>"
  VOUTP_ACCLevelMem12_enum/1 -> Data Type Conversion263/1
  VOUTP_ACCLevelMem34_enum/1 -> Data Type Conversion264/1
  VOUTP_ACCLevelMem57_enum/1 -> Data Type Conversion265/1
  Data Type Conversion263/1 -> Mux/238
  Data Type Conversion264/1 -> Mux/239
  Data Type Conversion265/1 -> Mux/240
  VOUTP_ModelVersionChksum_raw/1 -> Data Type Conversion267/1
  VOUTP_ModelVersion_raw/1 -> Data Type Conversion266/1
  Data Type Conversion266/1 -> Mux/246
  Data Type Conversion267/1 -> Mux/247
  VOUTP_HMIKey6FuncSta_enum/1 -> Data Type Conversion784/1
  VOUTP_HMIKey3FuncSta_enum/1 -> Data Type Conversion781/1
  Data Type Conversion780/1 -> Mux/249
  Data Type Conversion779/1 -> Mux/248
  VOUTP_HMIKey2FuncSta_enum/1 -> Data Type Conversion780/1
  VOUTP_HMIKey1FuncSta_enum/1 -> Data Type Conversion779/1
  VOUTP_AutoWipHSpdENSta_flg/1 -> Data Type Conversion787/1
  VOUTP_HMIKey8FuncSta_enum/1 -> Data Type Conversion786/1
  VOUTP_HMIKey4FuncSta_enum/1 -> Data Type Conversion782/1
  Data Type Conversion787/1 -> Mux/256
  Data Type Conversion786/1 -> Mux/255
  Data Type Conversion782/1 -> Mux/251
  VOUTP_HMIKey7FuncSta_enum/1 -> Data Type Conversion785/1
  Data Type Conversion784/1 -> Mux/253
  Data Type Conversion783/1 -> Mux/252
  Data Type Conversion781/1 -> Mux/250
  VOUTP_HMIKey5FuncSta_enum/1 -> Data Type Conversion783/1
  Data Type Conversion785/1 -> Mux/254
  [HAL_NvmWriteData256BytesArray3_raw] -> Mux2/3
  [HAL_NvmWriteData256BytesArray2_raw] -> Mux2/2
  [HAL_NvmWriteData256BytesArray1_raw] -> Mux2/1
  [HAL_NvmWriteData256BytesArray4_raw] -> Mux2/4
  Mux2/1 -> HAL_NvmWriteData_raw/1
  Constant1/1 -> [HAL_NvmWriteData256BytesArray3_raw]
  Constant2/1 -> [HAL_NvmWriteData256BytesArray4_raw]
  Mux1/1 -> [HAL_NvmWriteData256BytesArray2_raw]
  VOUTP_AirIntenZone1MSet2_enum/1 -> Data Type Conversion268/1
  VOUTP_AirIntenZone1MSet3_enum/1 -> Data Type Conversion269/1
  VOUTP_AirIntenZone1MSet5_enum/1 -> Data Type Conversion271/1
  VOUTP_AirIntenZone1MSet4_enum/1 -> Data Type Conversion270/1
  VOUTP_AirIntenZone3MSet3_enum/1 -> Data Type Conversion274/1
  VOUTP_AirIntenZone3MSet4_enum/1 -> Data Type Conversion275/1
  VOUTP_AirIntenZone3MSet2_enum/1 -> Data Type Conversion273/1
  VOUTP_AirIntenZone1MSet7_enum/1 -> Data Type Conversion272/1
  VOUTP_LEVentModeStaSet457_enum/1 -> Data Type Conversion280/1
  VOUTP_REVentModeStaSet457_enum/1 -> Data Type Conversion281/1
  VOUTP_FDCTHCLEVentZStaSet3_enum/1 -> Data Type Conversion283/1
  VOUTP_FDCTHCLEVentZStaSet2_enum/1 -> Data Type Conversion282/1
  VOUTP_FDCFGSChStaSet457_enum/1 -> Data Type Conversion278/1
  VOUTP_FDCFGSAirIntStaSet457_enum/1 -> Data Type Conversion279/1
  VOUTP_AirIntenZone3MSet7_enum/1 -> Data Type Conversion277/1
  VOUTP_AirIntenZone3MSet5_enum/1 -> Data Type Conversion276/1
  VOUTP_FDCTHCLEVentZStaSet4_enum/1 -> Data Type Conversion284/1
  VOUTP_FDCTHCLEVentZStaSet5_enum/1 -> Data Type Conversion285/1
  VOUTP_FDCTHCCLEVentZStaSet2_enum/1 -> Data Type Conversion287/1
  VOUTP_FDCTHCLEVentZStaSet7_enum/1 -> Data Type Conversion286/1
  VOUTP_FDCTHCCLEVentZStaSet5_enum/1 -> Data Type Conversion290/1
  VOUTP_FDCTHCCLEVentZStaSet7_enum/1 -> Data Type Conversion291/1
  VOUTP_FDCTHCCLEVentZStaSet4_enum/1 -> Data Type Conversion289/1
  VOUTP_FDCTHCCLEVentZStaSet3_enum/1 -> Data Type Conversion288/1
  VOUTP_FDCTHCREVentYStaSet2_enum/1 -> Data Type Conversion312/1
  VOUTP_FDCTHCREVentYStaSet3_enum/1 -> Data Type Conversion313/1
  VOUTP_FDCTHCREVentYStaSet5_enum/1 -> Data Type Conversion315/1
  VOUTP_FDCTHCREVentYStaSet4_enum/1 -> Data Type Conversion314/1
  VOUTP_FDCTHCCLEVentYStaSet5_enum/1 -> Data Type Conversion310/1
  VOUTP_FDCTHCCLEVentYStaSet7_enum/1 -> Data Type Conversion311/1
  VOUTP_FDCTHCCLEVentYStaSet4_enum/1 -> Data Type Conversion309/1
  VOUTP_FDCTHCCLEVentYStaSet3_enum/1 -> Data Type Conversion308/1
  VOUTP_FDCTHCCREVentZStaSet5_enum/1 -> Data Type Conversion300/1
  VOUTP_FDCTHCCREVentZStaSet7_enum/1 -> Data Type Conversion301/1
  VOUTP_FDCTHCLEVentYStaSet3_enum/1 -> Data Type Conversion303/1
  VOUTP_FDCTHCLEVentYStaSet2_enum/1 -> Data Type Conversion302/1
  VOUTP_FDCTHCLEVentYStaSet7_enum/1 -> Data Type Conversion306/1
  VOUTP_FDCTHCCLEVentYStaSet2_enum/1 -> Data Type Conversion307/1
  VOUTP_FDCTHCLEVentYStaSet5_enum/1 -> Data Type Conversion305/1
  VOUTP_FDCTHCLEVentYStaSet4_enum/1 -> Data Type Conversion304/1
  VOUTP_FDCTHCREVentZStaSet7_enum/1 -> Data Type Conversion296/1
  VOUTP_FDCTHCCREVentZStaSet2_enum/1 -> Data Type Conversion297/1
  VOUTP_FDCTHCCREVentZStaSet4_enum/1 -> Data Type Conversion299/1
  VOUTP_FDCTHCCREVentZStaSet3_enum/1 -> Data Type Conversion298/1
  VOUTP_FDCTHCREVentZStaSet4_enum/1 -> Data Type Conversion294/1
  VOUTP_FDCTHCREVentZStaSet5_enum/1 -> Data Type Conversion295/1
  VOUTP_FDCTHCREVentZStaSet3_enum/1 -> Data Type Conversion293/1
  VOUTP_FDCTHCREVentZStaSet2_enum/1 -> Data Type Conversion292/1
  VOUTP_FDCTHCREVentYStaSet7_enum/1 -> Data Type Conversion316/1
  VOUTP_FDCTHCCREVentYStaSet2_enum/1 -> Data Type Conversion317/1
  VOUTP_FDCTHCCREVentYStaSet4_enum/1 -> Data Type Conversion319/1
  VOUTP_FDCTHCCREVentYStaSet3_enum/1 -> Data Type Conversion318/1
  VOUTP_FDCTHCCREVentYStaSet5_enum/1 -> Data Type Conversion320/1
  VOUTP_FDCTHCCREVentYStaSet7_enum/1 -> Data Type Conversion321/1
  VOUTP_SettempZon1Set2_enum/1 -> Data Type Conversion323/1
  VOUTP_ACModeSet457_enum/1 -> Data Type Conversion322/1
  VOUTP_SettempZon1Set5_enum/1 -> Data Type Conversion326/1
  VOUTP_SettempZon1Set7_enum/1 -> Data Type Conversion327/1
  VOUTP_SettempZon1Set4_enum/1 -> Data Type Conversion325/1
  VOUTP_SettempZon1Set3_enum/1 -> Data Type Conversion324/1
  Data Type Conversion268/1 -> Mux1/1
  Data Type Conversion269/1 -> Mux1/2
  Data Type Conversion270/1 -> Mux1/3
  Data Type Conversion271/1 -> Mux1/4
  Data Type Conversion272/1 -> Mux1/5
  Data Type Conversion273/1 -> Mux1/6
  Data Type Conversion274/1 -> Mux1/7
  Data Type Conversion275/1 -> Mux1/8
  Data Type Conversion276/1 -> Mux1/9
  Data Type Conversion277/1 -> Mux1/10
  Data Type Conversion278/1 -> Mux1/11
  Data Type Conversion279/1 -> Mux1/12
  Data Type Conversion280/1 -> Mux1/13
  Data Type Conversion281/1 -> Mux1/14
  Data Type Conversion282/1 -> Mux1/15
  Data Type Conversion283/1 -> Mux1/16
  Data Type Conversion284/1 -> Mux1/17
  Data Type Conversion285/1 -> Mux1/18
  Data Type Conversion286/1 -> Mux1/19
  Data Type Conversion287/1 -> Mux1/20
  Data Type Conversion288/1 -> Mux1/21
  Data Type Conversion289/1 -> Mux1/22
  Data Type Conversion290/1 -> Mux1/23
  Data Type Conversion291/1 -> Mux1/24
  Data Type Conversion292/1 -> Mux1/25
  Data Type Conversion293/1 -> Mux1/26
  Data Type Conversion294/1 -> Mux1/27
  Data Type Conversion295/1 -> Mux1/28
  Data Type Conversion296/1 -> Mux1/29
  Data Type Conversion297/1 -> Mux1/30
  Data Type Conversion298/1 -> Mux1/31
  Data Type Conversion299/1 -> Mux1/32
  Data Type Conversion300/1 -> Mux1/33
  Data Type Conversion301/1 -> Mux1/34
  Data Type Conversion302/1 -> Mux1/35
  Data Type Conversion303/1 -> Mux1/36
  Data Type Conversion304/1 -> Mux1/37
  Data Type Conversion305/1 -> Mux1/38
  Data Type Conversion306/1 -> Mux1/39
  Data Type Conversion307/1 -> Mux1/40
  Data Type Conversion308/1 -> Mux1/41
  Data Type Conversion309/1 -> Mux1/42
  Data Type Conversion310/1 -> Mux1/43
  Data Type Conversion311/1 -> Mux1/44
  Data Type Conversion312/1 -> Mux1/45
  Data Type Conversion313/1 -> Mux1/46
  Data Type Conversion314/1 -> Mux1/47
  Data Type Conversion315/1 -> Mux1/48
  Data Type Conversion316/1 -> Mux1/49
  Data Type Conversion317/1 -> Mux1/50
  Data Type Conversion318/1 -> Mux1/51
  Data Type Conversion319/1 -> Mux1/52
  Data Type Conversion320/1 -> Mux1/53
  Data Type Conversion321/1 -> Mux1/54
  Data Type Conversion322/1 -> Mux1/55
  Data Type Conversion323/1 -> Mux1/56
  Data Type Conversion324/1 -> Mux1/57
  Data Type Conversion325/1 -> Mux1/58
  Data Type Conversion326/1 -> Mux1/59
  Data Type Conversion327/1 -> Mux1/60
  Ground2/1 -> Mux1/63
  Ground3/1 -> Mux1/64
  Ground4/1 -> Mux1/65
  Ground5/1 -> Mux1/66
  Ground6/1 -> Mux1/67
  Ground7/1 -> Mux1/68
  Ground8/1 -> Mux1/69
  Ground9/1 -> Mux1/70
  Ground10/1 -> Mux1/71
  Ground11/1 -> Mux1/72
  Ground12/1 -> Mux1/73
  Ground13/1 -> Mux1/74
  Ground14/1 -> Mux1/75
  Ground15/1 -> Mux1/76
  Ground16/1 -> Mux1/77
  Ground17/1 -> Mux1/78
  Ground24/1 -> Mux1/79
  Ground25/1 -> Mux1/80
  Ground26/1 -> Mux1/81
  Ground27/1 -> Mux1/82
  Ground28/1 -> Mux1/83
  Ground29/1 -> Mux1/84
  Ground30/1 -> Mux1/85
  Ground31/1 -> Mux1/86
  Ground18/1 -> Mux1/87
  Ground19/1 -> Mux1/88
  Ground20/1 -> Mux1/89
  Ground21/1 -> Mux1/90
  Ground22/1 -> Mux1/91
  Ground23/1 -> Mux1/92
  Ground32/1 -> Mux1/93
  Ground43/1 -> Mux1/94
  Ground54/1 -> Mux1/95
  Ground57/1 -> Mux1/96
  Ground58/1 -> Mux1/97
  Ground59/1 -> Mux1/98
  Ground60/1 -> Mux1/99
  Ground61/1 -> Mux1/100
  Ground62/1 -> Mux1/101
  Ground33/1 -> Mux1/102
  Ground34/1 -> Mux1/103
  Ground35/1 -> Mux1/104
  Ground36/1 -> Mux1/105
  Ground37/1 -> Mux1/106
  Ground38/1 -> Mux1/107
  Ground39/1 -> Mux1/108
  Ground40/1 -> Mux1/109
  Ground48/1 -> Mux1/110
  Ground49/1 -> Mux1/111
  Ground50/1 -> Mux1/112
  Ground51/1 -> Mux1/113
  Ground52/1 -> Mux1/114
  Ground53/1 -> Mux1/115
  Ground55/1 -> Mux1/116
  Ground56/1 -> Mux1/117
  Ground41/1 -> Mux1/118
  Ground42/1 -> Mux1/119
  Ground44/1 -> Mux1/120
  Ground45/1 -> Mux1/121
  Ground46/1 -> Mux1/122
  Ground47/1 -> Mux1/123
  Ground73/1 -> Mux1/124
  Ground84/1 -> Mux1/125
  Ground95/1 -> Mux1/126
  Ground106/1 -> Mux1/127
  Ground117/1 -> Mux1/128
  Ground121/1 -> Mux1/129
  Ground122/1 -> Mux1/130
  Ground123/1 -> Mux1/131
  Ground63/1 -> Mux1/132
  Ground64/1 -> Mux1/133
  Ground65/1 -> Mux1/134
  Ground66/1 -> Mux1/135
  Ground67/1 -> Mux1/136
  Ground68/1 -> Mux1/137
  Ground69/1 -> Mux1/138
  Ground70/1 -> Mux1/139
  Ground78/1 -> Mux1/140
  Ground79/1 -> Mux1/141
  Ground80/1 -> Mux1/142
  Ground81/1 -> Mux1/143
  Ground82/1 -> Mux1/144
  Ground83/1 -> Mux1/145
  Ground85/1 -> Mux1/146
  Ground86/1 -> Mux1/147
  Ground71/1 -> Mux1/148
  Ground72/1 -> Mux1/149
  Ground74/1 -> Mux1/150
  Ground75/1 -> Mux1/151
  Ground76/1 -> Mux1/152
  Ground77/1 -> Mux1/153
  Ground87/1 -> Mux1/154
  Ground99/1 -> Mux1/155
  Ground111/1 -> Mux1/156
  Ground114/1 -> Mux1/157
  Ground115/1 -> Mux1/158
  Ground116/1 -> Mux1/159
  Ground118/1 -> Mux1/160
  Ground119/1 -> Mux1/161
  Ground120/1 -> Mux1/162
  Ground88/1 -> Mux1/163
  Ground89/1 -> Mux1/164
  Ground90/1 -> Mux1/165
  Ground91/1 -> Mux1/166
  Ground92/1 -> Mux1/167
  Ground93/1 -> Mux1/168
  Ground94/1 -> Mux1/169
  Ground96/1 -> Mux1/170
  Ground104/1 -> Mux1/171
  Ground105/1 -> Mux1/172
  Ground107/1 -> Mux1/173
  Ground108/1 -> Mux1/174
  Ground109/1 -> Mux1/175
  Ground110/1 -> Mux1/176
  Ground112/1 -> Mux1/177
  Ground113/1 -> Mux1/178
  Ground97/1 -> Mux1/179
  Ground98/1 -> Mux1/180
  Ground100/1 -> Mux1/181
  Ground101/1 -> Mux1/182
  Ground102/1 -> Mux1/183
  Ground103/1 -> Mux1/184
  Ground158/1 -> Mux1/185
  Ground169/1 -> Mux1/186
  Ground180/1 -> Mux1/187
  Ground130/1 -> Mux1/188
  Ground141/1 -> Mux1/189
  Ground145/1 -> Mux1/190
  Ground146/1 -> Mux1/191
  Ground147/1 -> Mux1/192
  Ground148/1 -> Mux1/193
  Ground149/1 -> Mux1/194
  Ground150/1 -> Mux1/195
  Ground151/1 -> Mux1/196
  Ground152/1 -> Mux1/197
  Ground153/1 -> Mux1/198
  Ground154/1 -> Mux1/199
  Ground155/1 -> Mux1/200
  Ground163/1 -> Mux1/201
  Ground164/1 -> Mux1/202
  Ground165/1 -> Mux1/203
  Ground166/1 -> Mux1/204
  Ground167/1 -> Mux1/205
  Ground168/1 -> Mux1/206
  Ground170/1 -> Mux1/207
  Ground171/1 -> Mux1/208
  Ground156/1 -> Mux1/209
  Ground157/1 -> Mux1/210
  Ground159/1 -> Mux1/211
  Ground160/1 -> Mux1/212
  Ground161/1 -> Mux1/213
  Ground162/1 -> Mux1/214
  Ground172/1 -> Mux1/215
  Ground184/1 -> Mux1/216
  Ground135/1 -> Mux1/217
  Ground138/1 -> Mux1/218
  Ground139/1 -> Mux1/219
  Ground140/1 -> Mux1/220
  Ground142/1 -> Mux1/221
  Ground143/1 -> Mux1/222
  Ground144/1 -> Mux1/223
  Ground173/1 -> Mux1/224
  Ground174/1 -> Mux1/225
  Ground175/1 -> Mux1/226
  Ground176/1 -> Mux1/227
  Ground177/1 -> Mux1/228
  Ground178/1 -> Mux1/229
  Ground179/1 -> Mux1/230
  Ground181/1 -> Mux1/231
  Ground128/1 -> Mux1/232
  Ground129/1 -> Mux1/233
  Ground131/1 -> Mux1/234
  Ground132/1 -> Mux1/235
  Ground133/1 -> Mux1/236
  Ground134/1 -> Mux1/237
  Ground136/1 -> Mux1/238
  Ground137/1 -> Mux1/239
  Ground182/1 -> Mux1/240
  Ground183/1 -> Mux1/241
  Ground124/1 -> Mux1/242
  Ground125/1 -> Mux1/243
  Ground126/1 -> Mux1/244
  Ground127/1 -> Mux1/245
  Ground195/1 -> Mux1/256
  Ground189/1 -> Mux1/246
  Ground190/1 -> Mux1/247
  Ground191/1 -> Mux1/248
  Ground192/1 -> Mux1/249
  Ground193/1 -> Mux1/250
  Ground194/1 -> Mux1/251
  Ground185/1 -> Mux1/252
  Ground186/1 -> Mux1/253
  Ground187/1 -> Mux1/254
  Ground188/1 -> Mux1/255
  VOUTP_JudgeKeepUnlockZone_flg/1 -> Data Type Conversion328/1
  Data Type Conversion328/1 -> Mux1/61
  Data Type Conversion329/1 -> Mux1/62
  VOUTP_CLWinLockDrStaMem_enum/1 -> Data Type Conversion329/1
